simulink model "Animacion3d"  (Simulink 7.9)
settings: Solver=ode45  StartTime=0.0  StopTime=120.0  RelTol=1e-3
libraries: vrlib x1
settings Model: Creator=Henry  LastModifiedBy=Henry

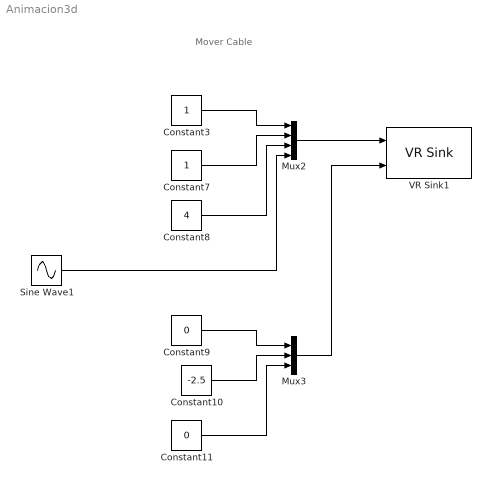
== system Animacion3d ==
  note: Mover Cable
  Constant10 : Constant  Value=-2.5
  Constant11 : Constant  Value=0
  Constant3 : Constant
  Constant7 : Constant
  Constant8 : Constant  Value=4
  Constant9 : Constant  Value=0
  Mux2 : Mux
  Mux3 : Mux  Inputs=3
  Sine Wave1 : Sin  Amplitude=10  Frequency=0.1  SampleTime=0
  VR Sink1 : vrlib/VR Sink  SampleTime=0.1  ViewEnable=on  RemoteChange=off  RemoteView=off  FieldsWritten=wire.rotation.4.1.1.double#wire.translation.3.1.1.double  WorldFileName=pendulo.wrl  AutoView=off  VideoDimensions=[]  AllowVariableSize=off
  wires:
  Mux2/1 -> VR Sink1/1
  Mux3/1 -> VR Sink1/2
  Constant3/1 -> Mux2/1
  Constant7/1 -> Mux2/2
  Constant8/1 -> Mux2/3
  Constant9/1 -> Mux3/1
  Constant10/1 -> Mux3/2
  Constant11/1 -> Mux3/3
  Sine Wave1/1 -> Mux2/4
